simulink model "Quadcopter_v3_full"  (R2021a)
settings: Solver=ode4  StartTime=0.0  StopTime=87  FixedStep=0.001  RelTol=1e-6
values from neighbouring files (symbols this model uses):
  mean_wind = [2.72 , 1.75, -0.006]    [main_run.m]    (also in main_run_5_1.m; param_est.m = [2.72 , 1.75, .006])
  q = X(7:10)    [EKF_without_wind.m]
  r = linspace(floor(nr*0.01)/nr,1,nr)    [main_run.m]    (also in main_run_5_1.m)
  w1 = w(1)    [EKF_without_wind.m]
  x0 = [0,0,0,1,0,0,0,-P.mean_wind,0,0,0]    [main_run.m]    (also in main_run_5_1.m)
  xref = [1,1,-8,1,0,0,0,-P.mean_wind]    [main_run.m]    (also in main_run_5_1.m)
undefined symbols (not defined in the file or in its folder): HDBK, MIL, Moderate, P, u1, v1
libraries: simulink x1, aerolibwind2 x1
(part 1 of 5)
settings Model: PauseTimes=2  Creator=lab  LastModifiedBy=lab
settings DebuggingCC: ReadBeforeWriteMsg=EnableAllAsWarning  WriteAfterWriteMsg=EnableAllAsWarning  WriteAfterReadMsg=EnableAllAsWarning  SFMachineParentedDataDiag=warning
settings SFSimCC: SimTargetLang=C++

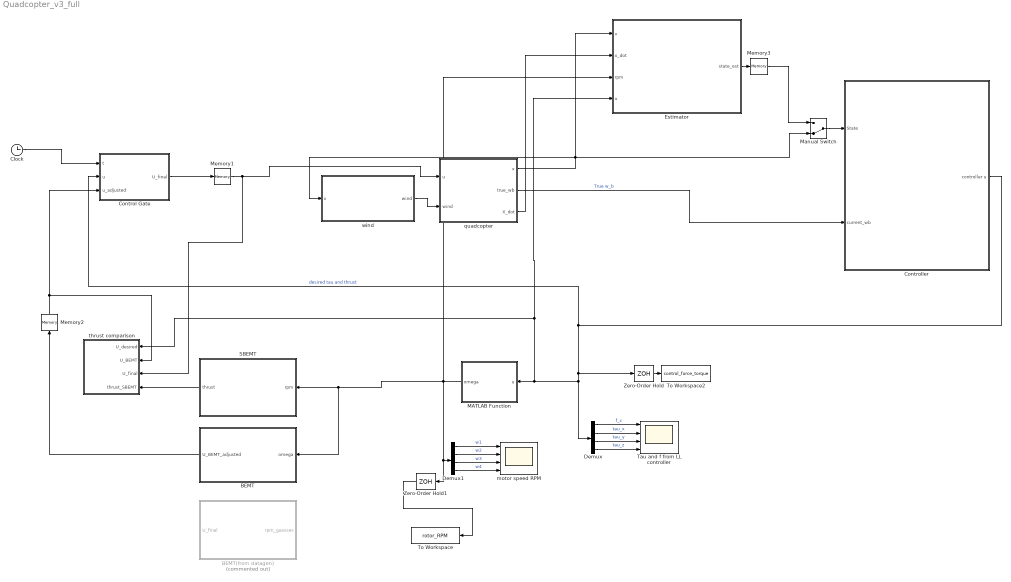
== system Quadcopter_v3_full ==
  BEMT : Subsystem
  BEMT(from datagen) : Subsystem  Commented=on
  Clock : Clock
  Control Gate : MATLAB Function  TreatAsAtomicUnit=on
  "Controller " : Subsystem
  Demux : Demux
  Demux1 : Demux
  Estimator : Subsystem
  MATLAB Function : MATLAB Function  TreatAsAtomicUnit=on
  Manual Switch : ManualSwitch  CurrentSetting=0
  Memory1 : Memory
  Memory2 : Memory
  Memory3 : Memory  InitialCondition=[0;0;0;1;0;0;0;0;0;0;0;0;0]
  SBEMT : Subsystem
  Tau and f from LL controller : Scope  NumInputPorts=4
  To Workspace : ToWorkspace  VariableName=rotor_RPM  SampleTime=-1
      settings: Save2DSignal=2-D array (concatenate along first dimension)
  To Workspace2 : ToWorkspace  VariableName=control_force_torque  SampleTime=-1
      settings: Save2DSignal=2-D array (concatenate along first dimension)
  Zero-Order Hold : ZeroOrderHold  SampleTime=0.01
  Zero-Order Hold1 : ZeroOrderHold  SampleTime=0.01
  motor speed RPM : Scope  NumInputPorts=4
  quadcopter : Subsystem
  thrust comparison : Subsystem
  wind : Subsystem
  wires:
  Zero-Order Hold/1 -> To Workspace2/1
  wind/1(wind) -> quadcopter/2(wind)
  Demux/1 -> Tau and f from LL controller/1  "f_c"
  Demux/2 -> Tau and f from LL controller/2  "tau_x"
  Demux/3 -> Tau and f from LL controller/3  "tau_y"
  Demux/4 -> Tau and f from LL controller/4  "tau_z"
  Demux1/2 -> motor speed RPM/2  "w2"
  Demux1/3 -> motor speed RPM/3  "w3"
  Demux1/4 -> motor speed RPM/4  "w4"
  Demux1/1 -> motor speed RPM/1  "w1"
  Zero-Order Hold1/1 -> To Workspace/1
  Control Gate/1(U_final) -> Memory1/1
  quadcopter/2(true_wb) -> "Controller "/2(current_wb)  "True w_b"
  quadcopter/3(X_dot) -> Estimator/2(x_dot)
  "Controller "/1(controller u) -> Demux/1, Estimator/4(u), thrust comparison/1(U_desired), MATLAB Function/1(u), Zero-Order Hold/1, Control Gate/2(u)  "desired tau and thrust"
  quadcopter/1(x) -> Estimator/1(x), Manual Switch/2, wind/1(x)
  MATLAB Function/1(omega) -> Estimator/3(rpm), BEMT/1(omega), SBEMT/1(rpm), Zero-Order Hold1/1, Demux1/1
  Memory1/1 -> thrust comparison/3(U_final), quadcopter/1(u)
  Clock/1 -> Control Gate/1(t)
  Memory2/1 -> thrust comparison/2(U_BEMT), Control Gate/3(u_adjusted)
  SBEMT/1(thrust) -> thrust comparison/4(thrust_SBEMT)
  BEMT/1(U_BEMT_adjusted) -> Memory2/1
  Estimator/1(state_est) -> Memory3/1
  Manual Switch/1 -> "Controller "/1(State)
  Memory3/1 -> Manual Switch/1

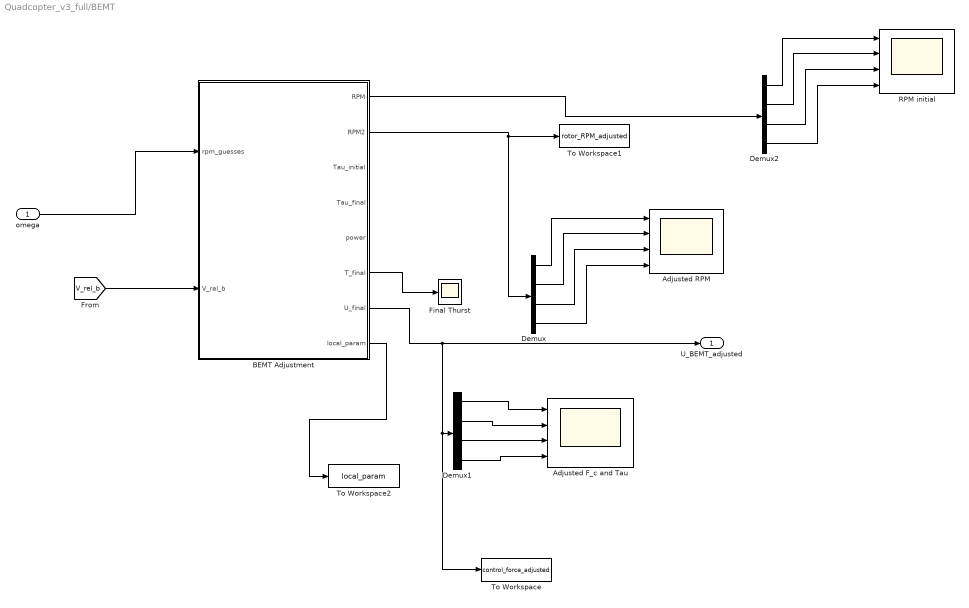
== system Quadcopter_v3_full/BEMT ==
  omega : Inport
  Adjusted F_c and Tau : Scope  NumInputPorts=4
  Adjusted RPM : Scope  NumInputPorts=4
  BEMT Adjustment : MATLAB Function  TreatAsAtomicUnit=on
  Demux : Demux
  Demux1 : Demux
  Demux2 : Demux
  Final Thurst : Scope
  RPM initial : Scope  NumInputPorts=4
  To Workspace : ToWorkspace  VariableName=control_force_adjusted  SampleTime=-1
      settings: Save2DSignal=2-D array (concatenate along first dimension)
  To Workspace1 : ToWorkspace  VariableName=rotor_RPM_adjusted  SampleTime=-1
      settings: Save2DSignal=2-D array (concatenate along first dimension)
  To Workspace2 : ToWorkspace  VariableName=local_param  SampleTime=-1
      settings: Save2DSignal=2-D array (concatenate along first dimension)
  U_BEMT_adjusted : Outport
  wires:
  omega/1 -> BEMT Adjustment/1(rpm_guesses)
  [V_rel_b] -> BEMT Adjustment/2(V_rel_b)
  BEMT Adjustment/2(RPM2) -> Demux/1, To Workspace1/1
  Demux/1 -> Adjusted RPM/1
  Demux/2 -> Adjusted RPM/2
  Demux/3 -> Adjusted RPM/3
  Demux/4 -> Adjusted RPM/4
  BEMT Adjustment/6(T_final) -> Final Thurst/1
  BEMT Adjustment/7(U_final) -> To Workspace/1, Demux1/1, U_BEMT_adjusted/1
  Demux1/1 -> Adjusted F_c and Tau/1
  Demux1/2 -> Adjusted F_c and Tau/2
  Demux1/3 -> Adjusted F_c and Tau/3
  Demux1/4 -> Adjusted F_c and Tau/4
  Demux2/1 -> RPM initial/1
  Demux2/4 -> RPM initial/4
  Demux2/3 -> RPM initial/3
  Demux2/2 -> RPM initial/2
  BEMT Adjustment/1(RPM) -> Demux2/1
  BEMT Adjustment/8(local_param) -> To Workspace2/1

== system Quadcopter_v3_full/BEMT(from datagen) ==
  rpm_guesses : Inport
  MATLAB Function1 : MATLAB Function  TreatAsAtomicUnit=on
  U_final : Outport
  wires:
  [V_rel_b] -> MATLAB Function1/2(V_rel_b)
  rpm_guesses/1 -> MATLAB Function1/1(rpm_guesses)
  MATLAB Function1/1(U_final) -> U_final/1

== system Quadcopter_v3_full/Controller  ==
  State : Inport
  current_wb : Inport  Port=2
  High Level Controller : Subsystem
  Low-Level Controller : Subsystem
      settings: PortSchema="{\"entries\":[{\"content\":{\"sides\":[{\"content\":{\"connectorIds\":[\"In1\"]},\"type\":\"ConnectorPlacement.EquallySpacedRectSide\",\"uuid\":\"a33d16ce-9843-4a8f-a539-e48e55dea327\"},{\"content\":{\"connectorIds\":[\"Out1\"],\"side\":\"RIGHT\"},\"type\":\"ConnectorPlacement.EquallySpacedRectSide\",\"uuid\":\"666ca801-6962-4f07-8037-ca18b43ecb76\"},{\"content\":{\"connectorIds\":[\"In2\"],\"side\":\"TOP\"},\"type\":\"ConnectorPlacement.EquallySpacedRectSide\",\"uuid\":\"a74aa88d-4aa1-42f8-8d8c-456156c6c0a0\"}]},\"type\":\"ConnectorPlacement.EquallySpacedConnector\",\"uuid\":\"b57d0f88-2cf0-4e3b-827d-8395103e5920\"}],\"packageUris\":[\"http://schema.mathworks.com/mf0/Connector/R2020b\"],\"version\":\"1.0\"}"
  To Workspace1 : ToWorkspace  VariableName=controller_omega  SampleTime=-1
      settings: Save2DSignal=2-D array (concatenate along first dimension)
  To Workspace5 : ToWorkspace  VariableName=states  SampleTime=-1
      settings: Save2DSignal=2-D array (concatenate along first dimension)
  Zero-Order Hold1 : ZeroOrderHold  SampleTime=0.01
  Zero-Order Hold2 : ZeroOrderHold  SampleTime=0.01
  controller u : Outport
  wires:
  State/1 -> High Level Controller/1(State), Zero-Order Hold2/1
  High Level Controller/1(" wx,wy,wz, f_c") -> Low-Level Controller/2(desired), Zero-Order Hold1/1  "desired w_b"
  current_wb/1 -> Low-Level Controller/1(prev_wb)
  Low-Level Controller/1(controller u) -> controller u/1  "desired tau and thrust"
  Zero-Order Hold2/1 -> To Workspace5/1
  Zero-Order Hold1/1 -> To Workspace1/1

== system Quadcopter_v3_full/Estimator ==
  x : Inport
  x_dot : Inport  Port=2
  rpm : Inport  Port=3
  u : Inport  Port=4
  Estimator : Subsystem
  To Workspace : ToWorkspace  VariableName=state_estimate  SampleTime=-1
      settings: Save2DSignal=2-D array (concatenate along first dimension)
  sensors : Subsystem
  state_est_aug : MATLAB Function  TreatAsAtomicUnit=on
  state_est : Outport
  wires:
  x/1 -> Estimator/5(X), sensors/1(x)
  sensors/1(GPS) -> Estimator/1(GPS)
  sensors/3(B_b) -> Estimator/3(B_b)
  rpm/1 -> Estimator/4(rpm)
  x_dot/1 -> sensors/2(x_dot)
  sensors/2(Accel_Gyro) -> state_est_aug/2(accel_gyro), Estimator/2(Accel_Gyro)
  u/1 -> Estimator/6(f_c)
  Estimator/1(state_est) -> state_est_aug/1(states_est), To Workspace/1
  state_est_aug/1(y) -> state_est/1

== system Quadcopter_v3_full/SBEMT ==
  rpm : Inport
  Simplified BEMT : MATLAB Function  TreatAsAtomicUnit=on
  thrust : Outport
  wires:
  rpm/1 -> Simplified BEMT/2(rpm)
  Simplified BEMT/1(Y) -> thrust/1  "SBEM f_c"
  [V_rel_b] -> Simplified BEMT/1(V_rb)

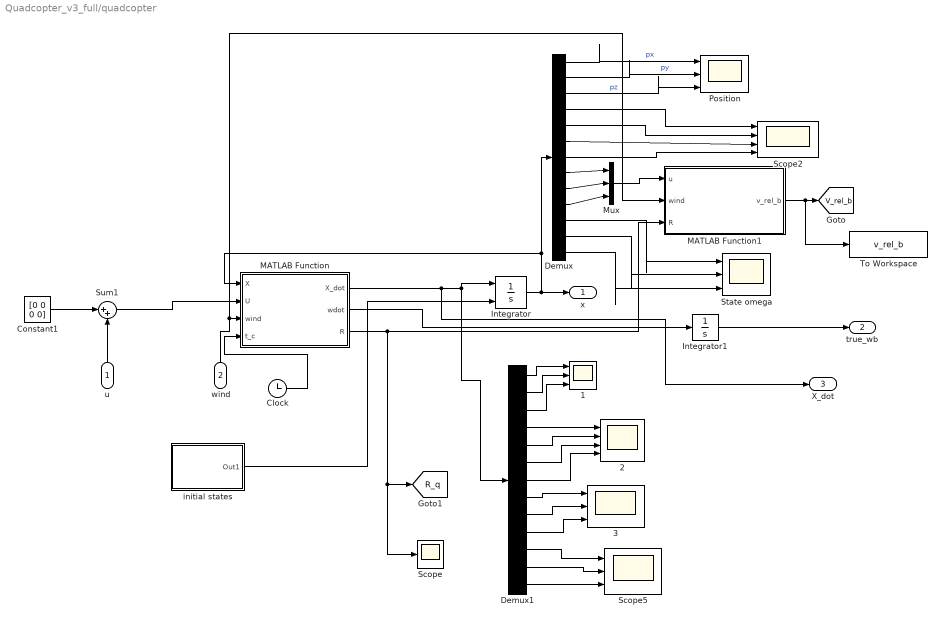
== system Quadcopter_v3_full/quadcopter ==
  u : Inport
  wind : Inport  Port=2
  1 : Scope  NumInputPorts=3
  2 : Scope  NumInputPorts=4
  3 : Scope  NumInputPorts=3
  Clock : Clock
  Constant1 : Constant  Value=[0 0 0 0]
  Demux : Demux  Outputs=13
  Demux1 : Demux  Outputs=13
  Integrator : Integrator  InitialConditionSource=external
  Integrator1 : Integrator  InitialCondition=[0,0,0]
  MATLAB Function : MATLAB Function  TreatAsAtomicUnit=on
  MATLAB Function1 : MATLAB Function  TreatAsAtomicUnit=on
  Mux : Mux  Inputs=3
  Position : Scope  NumInputPorts=3
  Scope : Scope
  Scope2 : Scope  NumInputPorts=4
  Scope5 : Scope  NumInputPorts=3
  State omega : Scope  NumInputPorts=3
  Sum1 : Sum  Inputs=|++
  To Workspace : ToWorkspace  VariableName=v_rel_b  SampleTime=-1
      settings: Save2DSignal=2-D array (concatenate along first dimension)
  initial states : Subsystem
  x : Outport
  true_wb : Outport  Port=2  OutDataTypeStr=double
  X_dot : Outport  Port=3
  tag scope: R_q=global, V_rel_b=global
  wires:
  Integrator/1 -> x/1, Demux/1, MATLAB Function/1(X)
  u/1 -> Sum1/2
  Sum1/1 -> MATLAB Function/2(U)
  Constant1/1 -> Sum1/1
  Demux1/6 -> 2/3
  Demux1/2 -> 1/2
  Demux1/5 -> 2/2
  Demux1/4 -> 2/1
  Demux1/3 -> 1/3
  Demux1/1 -> 1/1
  MATLAB Function/1(X_dot) -> X_dot/1, Integrator/1, Demux1/1
  wind/1 -> MATLAB Function1/2(wind), MATLAB Function/3(wind)
  initial states/1(Out1) -> Integrator/2
  Demux1/7 -> 2/4
  Demux1/8 -> 3/1
  Demux1/9 -> 3/2
  Demux1/10 -> 3/3
  Demux/1 -> Position/1  "px"
  Demux/2 -> Position/2  "py"
  Demux/3 -> Position/3  "pz"
  Demux/4 -> Scope2/1
  Demux/5 -> Scope2/2
  Demux/6 -> Scope2/3
  Demux/7 -> Scope2/4
  Demux1/11 -> Scope5/1
  Demux1/12 -> Scope5/2
  Demux1/13 -> Scope5/3
  MATLAB Function/2(wdot) -> Integrator1/1
  Demux/11 -> State omega/1
  Demux/12 -> State omega/2
  Demux/13 -> State omega/3
  Integrator1/1 -> true_wb/1
  Demux/8 -> Mux/1
  Demux/9 -> Mux/2
  Demux/10 -> Mux/3
  Mux/1 -> MATLAB Function1/1(u)
  MATLAB Function1/1(v_rel_b) -> To Workspace/1, [V_rel_b]
  MATLAB Function/3(R) -> Scope/1, [R_q], MATLAB Function1/3(R)
  Clock/1 -> MATLAB Function/4(t_c)

== system Quadcopter_v3_full/thrust comparison ==
  U_desired : Inport
  U_BEMT : Inport  Port=2
  U_final : Inport  Port=3
  thrust_SBEMT : Inport  Port=4
  Add : Sum  Inputs=+-
  Demux : Demux
  Demux1 : Demux
  Demux2 : Demux
  Scope : Scope  NumInputPorts=4
  Scope1 : Scope
  To Workspace : ToWorkspace  VariableName=thrust_desired  SampleTime=-1
      settings: Save2DSignal=2-D array (concatenate along first dimension)
  To Workspace1 : ToWorkspace  VariableName=thrust_BEMT  SampleTime=-1
      settings: Save2DSignal=2-D array (concatenate along first dimension)
  To Workspace2 : ToWorkspace  VariableName=thrust_final  SampleTime=-1
      settings: Save2DSignal=2-D array (concatenate along first dimension)
  To Workspace3 : ToWorkspace  VariableName=thrust_SBEMT  SampleTime=-1
      settings: Save2DSignal=2-D array (concatenate along first dimension)
  wires:
  U_desired/1 -> Demux/1
  U_BEMT/1 -> Demux1/1
  U_final/1 -> Demux2/1
  Demux/1 -> To Workspace/1, Scope/1  "thrust_desired"
  Demux1/1 -> To Workspace1/1, Scope/2  "thrust_BEMT"
  Demux2/1 -> Add/2, To Workspace2/1, Scope/3  "thrust_final"
  thrust_SBEMT/1 -> Add/1, To Workspace3/1, Scope/4  "thrust_SBEMT"
  Add/1 -> Scope1/1

== system Quadcopter_v3_full/wind ==
  x : Inport
  Constant_Wind : Subsystem
  Demux : Demux  Outputs=3
  Dryden Wind : Subsystem  Commented=on
  LES_wind : Subsystem  Commented=on
  Manual Switch : ManualSwitch
  To Workspace4 : ToWorkspace  VariableName=Wind  SampleTime=-1
      settings: Save2DSignal=2-D array (concatenate along first dimension)
  Zero-Order Hold1 : ZeroOrderHold  SampleTime=0.01
  sinusoidal_wind : Subsystem  Commented=on
  wind_vel : Scope  NumInputPorts=3
  wind : Outport
  wires:
  Manual Switch/1 -> Zero-Order Hold1/1, Demux/1, wind/1
  Constant_Wind/1(y) -> Manual Switch/1
  Zero-Order Hold1/1 -> To Workspace4/1
  LES_wind/1(Out1) -> Manual Switch/2
  x/1 -> LES_wind/1(x)
  Demux/1 -> wind_vel/1
  Demux/2 -> wind_vel/2
  Demux/3 -> wind_vel/3

== system Quadcopter_v3_full/Controller /High Level Controller ==
  State : Inport
  Clock : Clock
  Demux : Demux
  RS Controller : MATLAB Function  InitFcn="run(\"get_finitegain.m\")"  TreatAsAtomicUnit=on  SystemSampleTime=.05
  omega and fc from HL controller : Scope  NumInputPorts=4
  trajectory : Subsystem
  " wx,wy,wz, f_c" : Outport
  wires:
  RS Controller/1(y) -> " wx,wy,wz, f_c"/1, Demux/1
  trajectory/1(Out1) -> RS Controller/2(r)
  Demux/4 -> omega and fc from HL controller/4  "f_c"
  Demux/2 -> omega and fc from HL controller/2  "wy"
  Demux/1 -> omega and fc from HL controller/1  "wx"
  Demux/3 -> omega and fc from HL controller/3  "wz"
  State/1 -> RS Controller/1(x), trajectory/1(X)
  Clock/1 -> RS Controller/3(t)

== system Quadcopter_v3_full/Controller /Low-Level Controller ==
  prev_wb : Inport
  desired : Inport  Port=2
  Low level controller : MATLAB Function  TreatAsAtomicUnit=on  SystemSampleTime=.005
  controller u : Outport
  wires:
  Low level controller/1(u) -> controller u/1
  desired/1 -> Low level controller/2(desired)
  prev_wb/1 -> Low level controller/1(true_u)

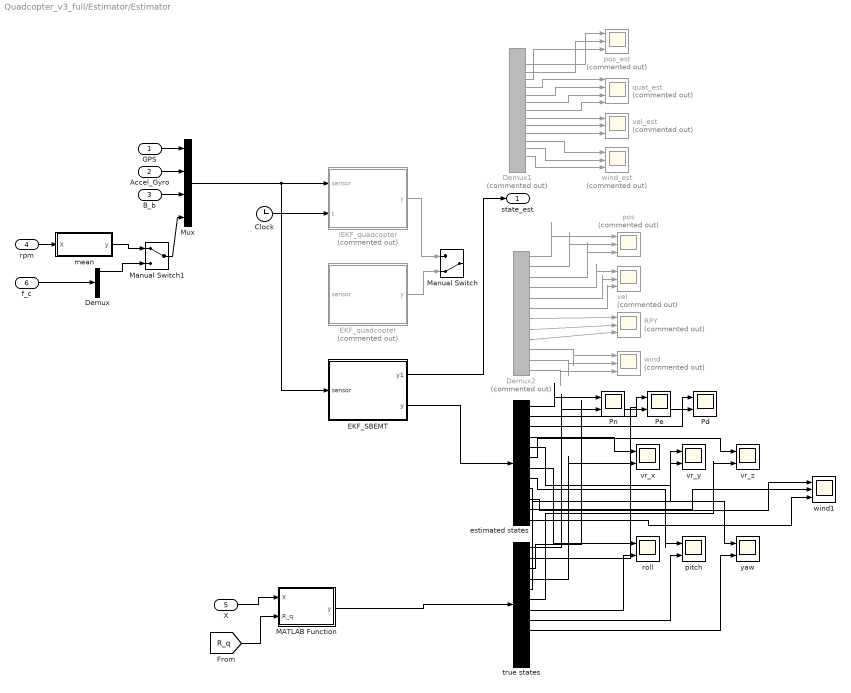
== system Quadcopter_v3_full/Estimator/Estimator ==
  GPS : Inport
  Accel_Gyro : Inport  Port=2
  B_b : Inport  Port=3
  rpm : Inport  Port=4
  X : Inport  Port=5
  f_c : Inport  Port=6
  Clock : Clock
  Demux : Demux
  Demux1 : Demux  Commented=on  Outputs=13
  Demux2 : Demux  Commented=on  Outputs=12
  EKF_SBEMT : MATLAB Function  InitFcn=addpath('quaternion_library');  TreatAsAtomicUnit=on  SystemSampleTime=0.01
  EKF_quadcopter : MATLAB Function  Commented=on  InitFcn=addpath('quaternion_library');  TreatAsAtomicUnit=on  SystemSampleTime=0.01
  IEKF_quadcopter : MATLAB Function  Commented=on  InitFcn=addpath('quaternion_library');  TreatAsAtomicUnit=on  SystemSampleTime=0.01
  MATLAB Function : MATLAB Function  TreatAsAtomicUnit=on
  Manual Switch : ManualSwitch  CurrentSetting=0
  Manual Switch1 : ManualSwitch
  Mux : Mux
  Pd : Scope  NumInputPorts=2
  Pe : Scope  NumInputPorts=2
  Pn : Scope  NumInputPorts=2
  RPY : Scope  Commented=on  NumInputPorts=3
  estimated states : Demux  Outputs=12
  mean : MATLAB Function  TreatAsAtomicUnit=on
  pitch : Scope  NumInputPorts=2
  pos : Scope  Commented=on  NumInputPorts=3
  pos_est : Scope  Commented=on  NumInputPorts=3
  quat_est : Scope  Commented=on  NumInputPorts=4
  roll : Scope  NumInputPorts=2
  true states : Demux  Outputs=12
  vel : Scope  Commented=on  NumInputPorts=3
  vel_est : Scope  Commented=on  NumInputPorts=3
  vr_x : Scope  NumInputPorts=2
  vr_y : Scope  NumInputPorts=2
  vr_z : Scope  NumInputPorts=2
  wind : Scope  Commented=on  NumInputPorts=3
  wind1 : Scope  NumInputPorts=3
  wind_est : Scope  Commented=on  NumInputPorts=3
  yaw : Scope  NumInputPorts=2
  state_est : Outport
  wires:
  GPS/1 -> Mux/1
  Accel_Gyro/1 -> Mux/2
  B_b/1 -> Mux/3
  rpm/1 -> mean/1(X)
  Demux1/1 -> pos_est/1
  Demux1/2 -> pos_est/2
  Demux1/3 -> pos_est/3
  Demux1/4 -> quat_est/1
  Demux1/5 -> quat_est/2
  Demux1/6 -> quat_est/3
  Demux1/7 -> quat_est/4
  Demux1/8 -> vel_est/1
  Demux1/9 -> vel_est/2
  Demux1/10 -> vel_est/3
  Demux1/11 -> wind_est/1
  Demux1/12 -> wind_est/2
  Demux1/13 -> wind_est/3
  Demux2/6 -> vel/3
  Demux2/5 -> vel/2
  Demux2/1 -> pos/1
  Demux2/2 -> pos/2
  Demux2/4 -> vel/1
  Demux2/3 -> pos/3
  Demux2/7 -> RPY/1
  Demux2/8 -> RPY/2
  Demux2/9 -> RPY/3
  Demux2/10 -> wind/1
  Demux2/11 -> wind/2
  Demux2/12 -> wind/3
  IEKF_quadcopter/1(y) -> Manual Switch/1
  X/1 -> MATLAB Function/1(X)
  estimated states/1 -> Pn/1
  true states/1 -> Pn/2
  estimated states/2 -> Pe/1
  true states/2 -> Pe/2
  estimated states/3 -> Pd/1
  true states/3 -> Pd/2
  estimated states/4 -> vr_x/1
  true states/4 -> vr_x/2
  estimated states/5 -> vr_y/1
  true states/5 -> vr_y/2
  estimated states/6 -> vr_z/1
  true states/6 -> vr_z/2
  estimated states/7 -> roll/1
  true states/7 -> roll/2
  estimated states/8 -> pitch/1
  true states/8 -> pitch/2
  estimated states/9 -> yaw/1
  true states/9 -> yaw/2
  MATLAB Function/1(y) -> true states/1
  estimated states/10 -> wind1/1
  estimated states/11 -> wind1/2
  estimated states/12 -> wind1/3
  Clock/1 -> IEKF_quadcopter/2(t)
  Mux/1 -> EKF_SBEMT/1(sensor), IEKF_quadcopter/1(sensor)
  Manual Switch1/1 -> Mux/4
  mean/1(y) -> Manual Switch1/1
  f_c/1 -> Demux/1
  Demux/1 -> Manual Switch1/2
  EKF_quadcopter/1(y) -> Manual Switch/2
  [R_q] -> MATLAB Function/2(R_q)
  EKF_SBEMT/2(y) -> estimated states/1
  EKF_SBEMT/1(y1) -> state_est/1

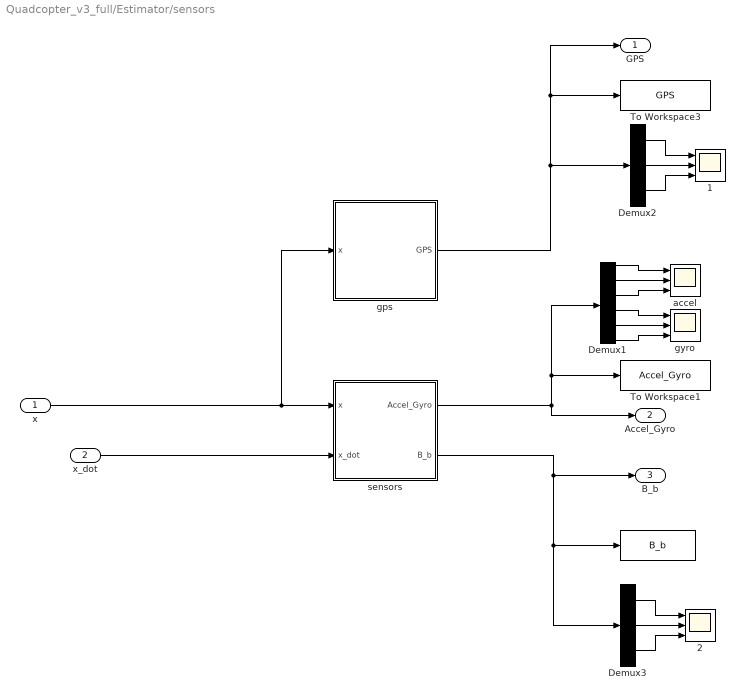
== system Quadcopter_v3_full/Estimator/sensors ==
  x : Inport
  x_dot : Inport  Port=2
  " " : ToWorkspace  VariableName=B_b  SampleTime=-1
      settings: Save2DSignal=2-D array (concatenate along first dimension)
  1 : Scope  NumInputPorts=3
  2 : Scope  NumInputPorts=3
  Demux1 : Demux  Outputs=6
  Demux2 : Demux  Outputs=3
  Demux3 : Demux  Outputs=3
  To Workspace1 : ToWorkspace  VariableName=Accel_Gyro  SampleTime=-1
      settings: Save2DSignal=2-D array (concatenate along first dimension)
  To Workspace3 : ToWorkspace  VariableName=GPS  SampleTime=-1
      settings: Save2DSignal=2-D array (concatenate along first dimension)
  accel : Scope  NumInputPorts=3
  gps : MATLAB Function  TreatAsAtomicUnit=on  SystemSampleTime=P.Ts_gps
  gyro : Scope  NumInputPorts=3
  sensors : MATLAB Function  TreatAsAtomicUnit=on  SystemSampleTime=P.Ts_gy_ac
  GPS : Outport
  Accel_Gyro : Outport  Port=2
  B_b : Outport  Port=3
  wires:
  Demux2/2 -> 1/2
  sensors/2(B_b) -> Demux3/1, " "/1, B_b/1
  Demux1/2 -> accel/2
  Demux3/2 -> 2/2
  Demux3/3 -> 2/3
  Demux2/3 -> 1/3
  x/1 -> sensors/1(x), gps/1(x)
  sensors/1(Accel_Gyro) -> Accel_Gyro/1, Demux1/1, To Workspace1/1
  gps/1(GPS) -> GPS/1, To Workspace3/1, Demux2/1
  Demux3/1 -> 2/1
  Demux1/3 -> accel/3
  Demux1/5 -> gyro/2
  Demux1/1 -> accel/1
  Demux1/4 -> gyro/1
  Demux1/6 -> gyro/3
  Demux2/1 -> 1/1
  x_dot/1 -> sensors/2(x_dot)

== system Quadcopter_v3_full/quadcopter/initial states ==
  Constant : Constant  Value=x0
  MATLAB Function1 : MATLAB Function  Commented=on  TreatAsAtomicUnit=on
  To Workspace4 : ToWorkspace  VariableName=X0  SampleTime=-1
  Out1 : Outport
  wires:
  Constant/1 -> To Workspace4/1, Out1/1

== system Quadcopter_v3_full/wind/Constant_Wind ==
  wind1 : Constant  Value=mean_wind
  y : Outport
  wires:
  wind1/1 -> y/1

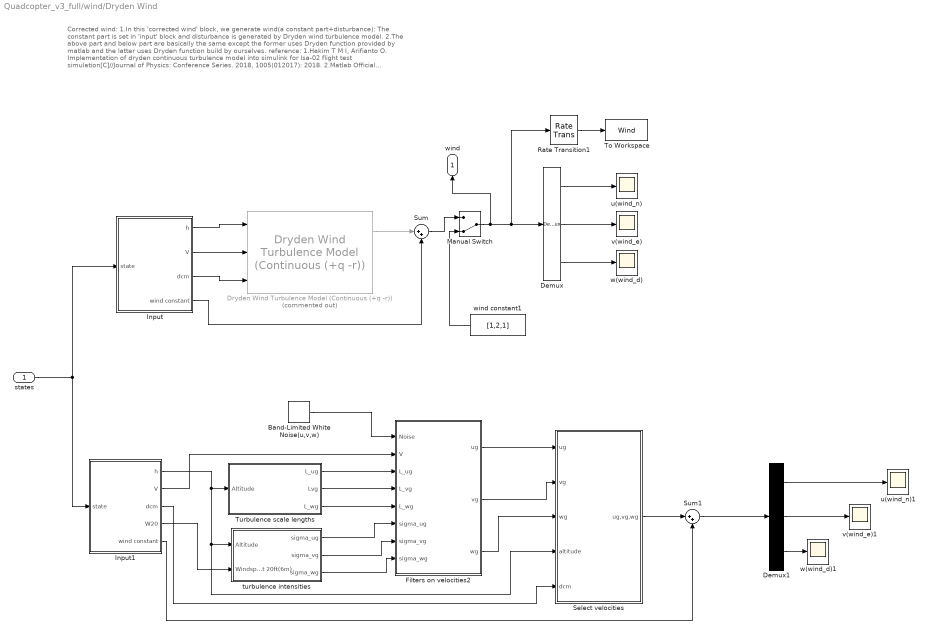
== system Quadcopter_v3_full/wind/Dryden Wind ==
  note: Corrected wind:
      | 1.In this 'corrected wind' block, we generate wind(a constant part+disturbance): The constant part is set in 'input' block and disturbance is generated by Dryden wind turbulence model.
      |
      | 2.The above part and below part are basically the same except the former uses Dryden function provided by matlab and the latter uses Dryden function build by ourselves.
      |
      | reference:
      | 1.Hakim T M I, Arifianto O. Implementation of dryden continuous turbulence model into simulink for lsa-02 flight test simulation[C]//Journal of Physics: Conference Series. 2018, 1005(012017): 2018.
      | 2.Matlab Official documents about Dryden Wind Turbulence Model
  states : Inport
  Band-Limited White Noise(u,v,w) : simulink/Sources/Band-Limited White Noise  Cov=[1 1 1]*pi  Ts=0.1  seed=[23341 23342 23343]
  Demux : Demux  Outputs=3
  Demux1 : Demux  Outputs=3
  Dryden Wind Turbulence Model (Continuous (+q -r)) : aerolibwind2/Dryden Wind Turbulence Model  (Continuous (+q -r))  Commented=on  units=Metric (MKS)  spec=MIL-HDBK-1797  model=Continuous Dryden (-q +r)  W20=15  Wdeg=45  TurbProb=10^-3 - Moderate  L_high=533.4  Wingspan=0.4  ts=0.1  Seed=[23341 23342 23343 23344]  T_on=on
  Filters on velocities2 : Subsystem
  Input : Subsystem
  Input1 : Subsystem
  Manual Switch : ManualSwitch  CurrentSetting=0
  Rate Transition1 : RateTransition  OutPortSampleTime=0.01
  Select velocities : Subsystem
  Sum : Sum  Inputs=|++
  Sum1 : Sum  Inputs=|++
  To Workspace : ToWorkspace  VariableName=Wind  SaveFormat=Timeseries  SampleTime=-1
  Turbulence scale lengths : Subsystem
  turbulence intensities : Subsystem
  u(wind_n) : Scope
  u(wind_n)1 : Scope
  v(wind_e) : Scope
  v(wind_e)1 : Scope
  w(wind_d) : Scope
  w(wind_d)1 : Scope
  wind constant1 : Constant  Value=[1,2,1]
  wind : Outport
  wires:
  Input/1(h) -> Dryden Wind Turbulence Model (Continuous (+q -r))/1
  Input/2(V) -> Dryden Wind Turbulence Model (Continuous (+q -r))/2
  Input/3(dcm) -> Dryden Wind Turbulence Model (Continuous (+q -r))/3
  states/1 -> Input/1(state), Input1/1(state)
  Dryden Wind Turbulence Model (Continuous (+q -r))/1 -> Sum/1
  Input1/1(h) -> Turbulence scale lengths/1(Altitude), turbulence intensities/1(Altitude), Select velocities/4(altitude)
  Input1/4(W20) -> turbulence intensities/2(Windspeed at 20ft(6m))
  turbulence intensities/2(sigma_vg) -> Filters on velocities2/7(sigma_vg)
  turbulence intensities/3(sigma_wg) -> Filters on velocities2/8(sigma_wg)
  Turbulence scale lengths/1(L_ug) -> Filters on velocities2/3(L_ug)
  Turbulence scale lengths/2(Lvg) -> Filters on velocities2/4(L_vg)
  Turbulence scale lengths/3(L_wg) -> Filters on velocities2/5(L_wg)
  Band-Limited White Noise(u,v,w)/1 -> Filters on velocities2/1(Noise)
  Input1/2(V) -> Filters on velocities2/2(V)
  turbulence intensities/1(sigma_ug) -> Filters on velocities2/6(sigma_ug)
  Filters on velocities2/1(ug) -> Select velocities/1(ug)
  Filters on velocities2/2(vg) -> Select velocities/2(vg)
  Filters on velocities2/3(wg) -> Select velocities/3(wg)
  Input1/3(dcm) -> Select velocities/5(dcm)
  Demux/1 -> u(wind_n)/1
  Demux/2 -> v(wind_e)/1
  Demux/3 -> w(wind_d)/1
  Input/4(wind constant) -> Sum/2
  Demux1/1 -> u(wind_n)1/1
  Demux1/2 -> v(wind_e)1/1
  Demux1/3 -> w(wind_d)1/1
  Input1/5(wind constant) -> Sum1/2
  Select velocities/1(ug,vg,wg) -> Sum1/1
  Sum1/1 -> Demux1/1
  Manual Switch/1 -> Rate Transition1/1, Demux/1, wind/1
  Sum/1 -> Manual Switch/1
  wind constant1/1 -> Manual Switch/2
  Rate Transition1/1 -> To Workspace/1

== system Quadcopter_v3_full/wind/LES_wind ==
  x : Inport
  Clock : Clock
  Constant : Constant  Value=u1
  Constant1 : Constant  Value=v1
  Constant2 : Constant  Value=w1
  From Workspace : FromWorkspace  Commented=on  VariableName=LES_wind_8m  SampleTime=-1
  From Workspace1 : FromWorkspace  VariableName=LES_wind  SampleTime=1
  MATLAB Function : MATLAB Function  TreatAsAtomicUnit=on
  Manual Switch1 : ManualSwitch
  Out1 : Outport
  wires:
  Manual Switch1/1 -> Out1/1
  x/1 -> MATLAB Function/1(x)
  Clock/1 -> MATLAB Function/2(t)
  Constant/1 -> MATLAB Function/3(u_wind)
  Constant1/1 -> MATLAB Function/4(v_wind)
  Constant2/1 -> MATLAB Function/5(w_wind)
  From Workspace1/1 -> Manual Switch1/1
  MATLAB Function/1(wind_vel) -> Manual Switch1/2

== system Quadcopter_v3_full/wind/sinusoidal_wind ==
  Clock : Clock
  From Workspace : FromWorkspace  VariableName=LES_wind_8m  SampleTime=-1
  Scope : Scope
  To Workspace4 : ToWorkspace  VariableName=Wind  SaveFormat=Timeseries  SampleTime=-1
  Zero-Order Hold1 : ZeroOrderHold  SampleTime=0.01
  sinusoidal part : MATLAB Function  TreatAsAtomicUnit=on
  y : Outport
  wires:
  From Workspace/1 -> sinusoidal part/1(LES)
  Clock/1 -> sinusoidal part/2(t)
  Zero-Order Hold1/1 -> To Workspace4/1
  sinusoidal part/1(y) -> Zero-Order Hold1/1, Scope/1, y/1

== system Quadcopter_v3_full/Controller /High Level Controller/trajectory ==
  X : Inport
  Clock : Clock
  "Desired Position, quat and velocity " : Constant  Value=xref
  MATLAB Function : MATLAB Function  TreatAsAtomicUnit=on
  Manual Switch : ManualSwitch  CurrentSetting=0
  circle_traj : MATLAB Function  Commented=on  TreatAsAtomicUnit=on
  squre_traj : MATLAB Function  Commented=on  TreatAsAtomicUnit=on
  Out1 : Outport
  wires:
  Manual Switch/1 -> Out1/1
  "Desired Position, quat and velocity "/1 -> Manual Switch/1
  X/1 -> squre_traj/1(X)
  Clock/1 -> MATLAB Function/1(t)
  MATLAB Function/1(xdes) -> Manual Switch/2

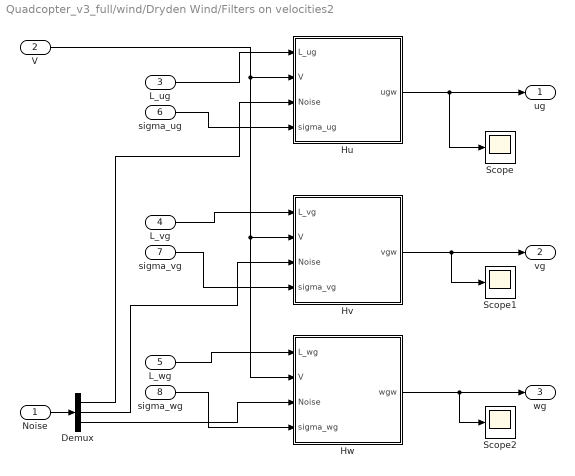
== system Quadcopter_v3_full/wind/Dryden Wind/Filters on velocities2 ==
  Noise : Inport
  V : Inport  Port=2
  L_ug : Inport  Port=3
  L_vg : Inport  Port=4
  L_wg : Inport  Port=5
  sigma_ug : Inport  Port=6
  sigma_vg : Inport  Port=7
  sigma_wg : Inport  Port=8
  Demux : Demux  Outputs=3
  Hu : Subsystem
  Hv : Subsystem
  Hw : Subsystem
  Scope : Scope
  Scope1 : Scope
  Scope2 : Scope
  ug : Outport
  vg : Outport  Port=2
  wg : Outport  Port=3
  wires:
  Noise/1 -> Demux/1
  V/1 -> Hw/2(V), Hv/2(V), Hu/2(V)
  L_ug/1 -> Hu/1(L_ug)
  sigma_ug/1 -> Hu/4(sigma_ug)
  Hu/1(ugw) -> Scope/1, ug/1
  L_vg/1 -> Hv/1(L_vg)
  sigma_vg/1 -> Hv/4(sigma_vg)
  Hv/1(vgw) -> Scope1/1, vg/1
  L_wg/1 -> Hw/1(L_wg)
  Demux/1 -> Hu/3(Noise)
  Demux/2 -> Hv/3(Noise)
  Demux/3 -> Hw/3(Noise)
  sigma_wg/1 -> Hw/4(sigma_wg)
  Hw/1(wgw) -> Scope2/1, wg/1

== system Quadcopter_v3_full/wind/Dryden Wind/Input ==
  state : Inport
  Abs : Abs
  DCM/rotation matrix : MATLAB Function  TreatAsAtomicUnit=on
  Demux : Demux  Outputs=12
  MATLAB Function : MATLAB Function  TreatAsAtomicUnit=on
  Mux : Mux  Inputs=9
  Mux1 : Mux  Inputs=3
  Scope : Scope
  Terminator : Terminator
  wind : Constant  Value=[0.1,0.1,0]
  h : Outport
  V : Outport  Port=2
  dcm : Outport  Port=3
  wind constant : Outport  Port=4
  wires:
  state/1 -> DCM/rotation matrix/1(x), Demux/1
  DCM/rotation matrix/1(R) -> dcm/1
  Mux/1 -> Terminator/1
  Demux/1 -> Mux/1
  MATLAB Function/1(V) -> Scope/1, V/1
  Demux/4 -> Mux1/1
  Demux/5 -> Mux1/2
  Demux/6 -> Mux1/3
  Demux/2 -> Mux/2
  Demux/3 -> Abs/1, Mux/3
  Demux/7 -> Mux/4
  Demux/8 -> Mux/5
  Demux/9 -> Mux/6
  Demux/10 -> Mux/7
  Demux/11 -> Mux/8
  Demux/12 -> Mux/9
  wind/1 -> wind constant/1, MATLAB Function/1(wind)
  Mux1/1 -> MATLAB Function/2(vel)
  Abs/1 -> h/1

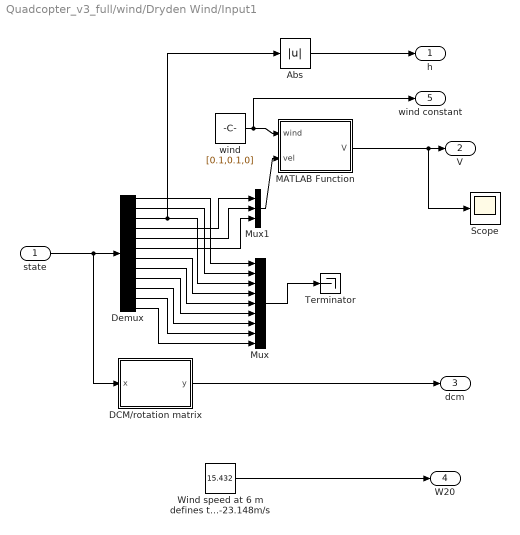
== system Quadcopter_v3_full/wind/Dryden Wind/Input1 ==
  state : Inport
  Abs : Abs
  DCM/rotation matrix : MATLAB Function  TreatAsAtomicUnit=on
  Demux : Demux  Outputs=12
  MATLAB Function : MATLAB Function  TreatAsAtomicUnit=on
  Mux : Mux  Inputs=9
  Mux1 : Mux  Inputs=3
  Scope : Scope
  Terminator : Terminator
  Wind speed at 6 m defines the low-altitude intensity (m/s) Light-7.716m/s Moderate-15.432m/s Severe-23.148m/s : Constant  Value=15.432
  wind : Constant  Value=[0.1,0.1,0]
  h : Outport
  V : Outport  Port=2
  dcm : Outport  Port=3
  W20 : Outport  Port=4
  wind constant : Outport  Port=5
  wires:
  state/1 -> DCM/rotation matrix/1(x), Demux/1
  DCM/rotation matrix/1(y) -> dcm/1
  Mux/1 -> Terminator/1
  Demux/1 -> Mux/1
  MATLAB Function/1(V) -> Scope/1, V/1
  Demux/4 -> Mux1/1
  Demux/5 -> Mux1/2
  Demux/6 -> Mux1/3
  Demux/2 -> Mux/2
  Demux/3 -> Abs/1, Mux/3
  Demux/7 -> Mux/4
  Demux/8 -> Mux/5
  Demux/9 -> Mux/6
  Demux/10 -> Mux/7
  Demux/11 -> Mux/8
  Demux/12 -> Mux/9
  wind/1 -> wind constant/1, MATLAB Function/1(wind)
  Mux1/1 -> MATLAB Function/2(vel)
  Wind speed at 6 m defines the low-altitude intensity (m/s) Light-7.716m/s Moderate-15.432m/s Severe-23.148m/s/1 -> W20/1
  Abs/1 -> h/1

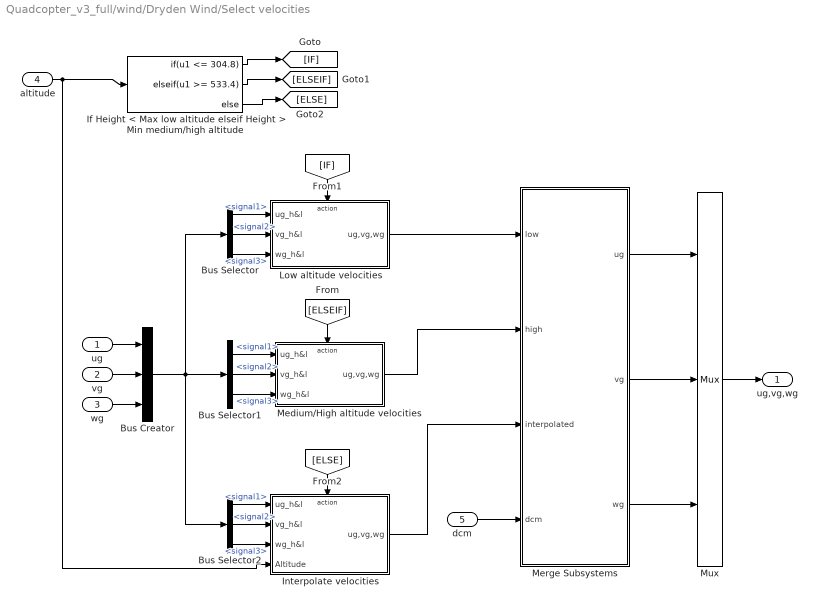
== system Quadcopter_v3_full/wind/Dryden Wind/Select velocities ==
  ug : Inport
  vg : Inport  Port=2
  wg : Inport  Port=3
  altitude : Inport  Port=4
  dcm : Inport  Port=5
  Bus Creator : BusCreator  Inputs=3
  Bus Selector : BusSelector  OutputSignals=signal1,signal2,signal3
  Bus Selector1 : BusSelector  OutputSignals=signal1,signal2,signal3
  Bus Selector2 : BusSelector  OutputSignals=signal1,signal2,signal3
  If Height < Max low altitude elseif Height > Min medium/high altitude : If  IfExpression=u1 <= 304.8  ElseIfExpressions=u1 >= 533.4
  Interpolate velocities : Subsystem  TreatAsAtomicUnit=on
  "Low altitude velocities " : Subsystem  TreatAsAtomicUnit=on
  Medium/High altitude velocities : Subsystem  TreatAsAtomicUnit=on
  Merge Subsystems : Subsystem
  Mux : Mux  Inputs=3
  ug,vg,wg : Outport
  wires:
  altitude/1 -> Interpolate velocities/4(Altitude), If Height < Max low altitude elseif Height > Min medium/high altitude/1
  If Height < Max low altitude elseif Height > Min medium/high altitude/1 -> [IF]
  If Height < Max low altitude elseif Height > Min medium/high altitude/2 -> [ELSEIF]
  [ELSEIF] -> Medium/High altitude velocities/Action
  "Low altitude velocities "/1(ug,vg,wg) -> Merge Subsystems/1(low)
  [IF] -> "Low altitude velocities "/Action
  Interpolate velocities/1(ug,vg,wg) -> Merge Subsystems/3(interpolated)
  [ELSE] -> Interpolate velocities/Action
  dcm/1 -> Merge Subsystems/4(dcm)
  vg/1 -> Bus Creator/2
  wg/1 -> Bus Creator/3
  ug/1 -> Bus Creator/1
  Bus Creator/1 -> Bus Selector2/1, Bus Selector1/1, Bus Selector/1
  Bus Selector2/1 -> Interpolate velocities/1(ug_h&l)  "<signal1>"
  Bus Selector2/2 -> Interpolate velocities/2(vg_h&l)  "<signal2>"
  Bus Selector2/3 -> Interpolate velocities/3(wg_h&l)  "<signal3>"
  Bus Selector/1 -> "Low altitude velocities "/1(ug_h&l)  "<signal1>"
  Bus Selector/2 -> "Low altitude velocities "/2(vg_h&l)  "<signal2>"
  Bus Selector/3 -> "Low altitude velocities "/3(wg_h&l)  "<signal3>"
  Bus Selector1/1 -> Medium/High altitude velocities/1(ug_h&l)  "<signal1>"
  Bus Selector1/2 -> Medium/High altitude velocities/2(vg_h&l)  "<signal2>"
  Bus Selector1/3 -> Medium/High altitude velocities/3(wg_h&l)  "<signal3>"
  If Height < Max low altitude elseif Height > Min medium/high altitude/3 -> [ELSE]
  Medium/High altitude velocities/1(ug,vg,wg) -> Merge Subsystems/2(high)
  Merge Subsystems/2(vg) -> Mux/2
  Merge Subsystems/1(ug) -> Mux/1
  Merge Subsystems/3(wg) -> Mux/3
  Mux/1 -> ug,vg,wg/1

== system Quadcopter_v3_full/wind/Dryden Wind/Turbulence scale lengths ==
  Altitude : Inport
  Low altitude scale length : Subsystem
  Medium/High altitude scale length : Subsystem
  Mux : Mux  Inputs=2
  Mux1 : Mux  Inputs=2
  Mux2 : Mux  Inputs=2
  L_ug : Outport
  Lvg : Outport  Port=2
  L_wg : Outport  Port=3
  wires:
  Medium/High altitude scale length/1(L_ug) -> Mux/2
  Altitude/1 -> Low altitude scale length/1(h)
  Low altitude scale length/3(L_wg) -> Mux2/1
  Low altitude scale length/2(Lvg) -> Mux1/1
  Mux1/1 -> Lvg/1
  Mux/1 -> L_ug/1
  Mux2/1 -> L_wg/1
  Medium/High altitude scale length/2(Lvg) -> Mux1/2
  Low altitude scale length/1(L_ug) -> Mux/1
  Medium/High altitude scale length/3(L_wg) -> Mux2/2

== system Quadcopter_v3_full/wind/Dryden Wind/turbulence intensities ==
  Altitude : Inport
  Windspeed at 20ft(6m) : Inport  Port=2
  High Altitude Intensity : Subsystem
  Low Altitude Intensity : Subsystem
  Mux : Mux  Inputs=2
  Mux1 : Mux  Inputs=2
  Mux2 : Mux  Inputs=2
  sigma_ug : Outport
  sigma_vg : Outport  Port=2
  sigma_wg : Outport  Port=3
  wires:
  Altitude/1 -> High Altitude Intensity/1(h), Low Altitude Intensity/1(h)
  Windspeed at 20ft(6m)/1 -> Low Altitude Intensity/2(Windspeed at 20ft(6m))
  Low Altitude Intensity/1(sigma_ug) -> Mux/1
  High Altitude Intensity/1(sigma_ug) -> Mux/2
  High Altitude Intensity/2(sigma_vg) -> Mux1/2
  Low Altitude Intensity/2(sigma_vg) -> Mux1/1
  High Altitude Intensity/3(sigma_wg) -> Mux2/2
  Low Altitude Intensity/3(sigma_wg) -> Mux2/1
  Mux1/1 -> sigma_vg/1
  Mux/1 -> sigma_ug/1
  Mux2/1 -> sigma_wg/1

== system Quadcopter_v3_full/wind/Dryden Wind/Filters on velocities2/Hu ==
  L_ug : Inport
  V : Inport  Port=2
  Noise : Inport  Port=3
  sigma_ug : Inport  Port=4
  (2/pi) : Gain  Gain=2/pi
  L_ug/V : Product  Inputs=*/
  Product : Product
  Product1 : Product
  Sqrt : Sqrt  SaturateOnIntegerOverflow=on
  Sum : Sum  Inputs=|+-
  ug_p : Integrator
  w : Product  Inputs=*/
  ugw : Outport
  wires:
  L_ug/1 -> L_ug/V/1
  V/1 -> L_ug/V/2
  L_ug/V/1 -> w/2, (2/pi)/1
  (2/pi)/1 -> Sqrt/1
  Sqrt/1 -> Product/1
  Noise/1 -> Product/2
  Product/1 -> Sum/1
  Sum/1 -> w/1
  w/1 -> ug_p/1
  ug_p/1 -> Sum/2, Product1/1
  sigma_ug/1 -> Product1/2
  Product1/1 -> ugw/1

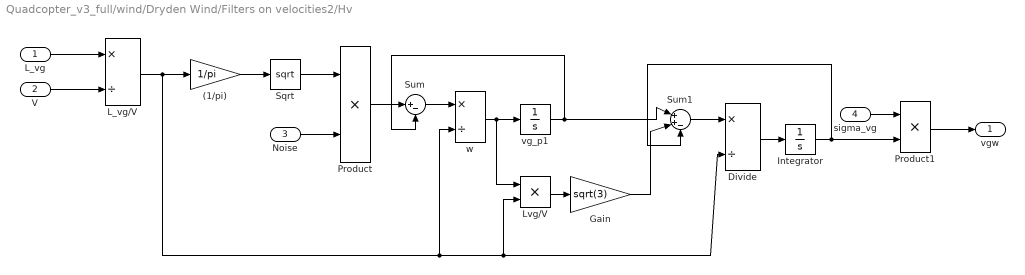
== system Quadcopter_v3_full/wind/Dryden Wind/Filters on velocities2/Hv ==
  L_vg : Inport
  V : Inport  Port=2
  Noise : Inport  Port=3
  sigma_vg : Inport  Port=4
  (1/pi) : Gain  Gain=1/pi
  Divide : Product  Inputs=*/
  Gain : Gain  Gain=sqrt(3)
  Integrator : Integrator
  L_vg/V : Product  Inputs=*/
  Lvg/V : Product
  Product : Product
  Product1 : Product
  Sqrt : Sqrt  SaturateOnIntegerOverflow=on
  Sum : Sum  Inputs=|+-
  Sum1 : Sum  Inputs=|++-
  vg_p1 : Integrator
  w : Product  Inputs=*/
  vgw : Outport
  wires:
  L_vg/1 -> L_vg/V/1
  V/1 -> L_vg/V/2
  L_vg/V/1 -> w/2, Lvg/V/2, Divide/2, (1/pi)/1
  (1/pi)/1 -> Sqrt/1
  Sqrt/1 -> Product/1
  Noise/1 -> Product/2
  Product/1 -> Sum/1
  Sum/1 -> w/1
  w/1 -> Lvg/V/1, vg_p1/1
  Lvg/V/1 -> Gain/1
  vg_p1/1 -> Sum1/1, Sum/2
  Gain/1 -> Sum1/2
  Sum1/1 -> Divide/1
  Divide/1 -> Integrator/1
  Integrator/1 -> Sum1/3, Product1/2
  Product1/1 -> vgw/1
  sigma_vg/1 -> Product1/1

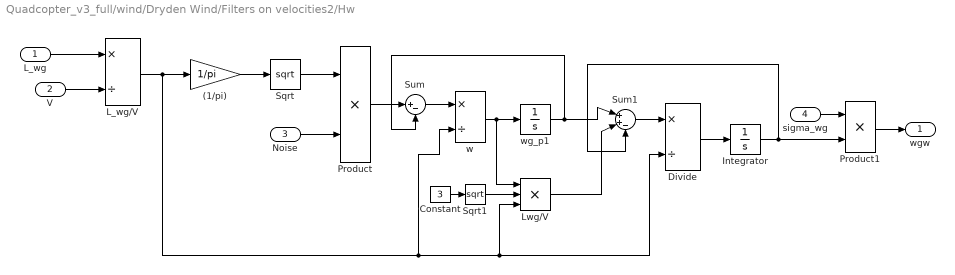
== system Quadcopter_v3_full/wind/Dryden Wind/Filters on velocities2/Hw ==
  L_wg : Inport
  V : Inport  Port=2
  Noise : Inport  Port=3
  sigma_wg : Inport  Port=4
  (1/pi) : Gain  Gain=1/pi
  Constant : Constant  Value=3
  Divide : Product  Inputs=*/
  Integrator : Integrator
  L_wg/V : Product  Inputs=*/
  Lwg/V : Product  Inputs=3
  Product : Product
  Product1 : Product
  Sqrt : Sqrt  SaturateOnIntegerOverflow=on
  Sqrt1 : Sqrt  SaturateOnIntegerOverflow=on
  Sum : Sum  Inputs=|+-
  Sum1 : Sum  Inputs=|++-
  w : Product  Inputs=*/
  wg_p1 : Integrator
  wgw : Outport
  wires:
  L_wg/1 -> L_wg/V/1
  V/1 -> L_wg/V/2
  L_wg/V/1 -> Lwg/V/3, Divide/2, w/2, (1/pi)/1
  (1/pi)/1 -> Sqrt/1
  Sqrt/1 -> Product/1
  Noise/1 -> Product/2
  Product/1 -> Sum/1
  Sum/1 -> w/1
  w/1 -> Lwg/V/1, wg_p1/1
  Lwg/V/1 -> Sum1/2
  wg_p1/1 -> Sum1/1, Sum/2
  Sum1/1 -> Divide/1
  Divide/1 -> Integrator/1
  Integrator/1 -> Product1/2, Sum1/3
  Product1/1 -> wgw/1
  sigma_wg/1 -> Product1/1
  Constant/1 -> Sqrt1/1
  Sqrt1/1 -> Lwg/V/2

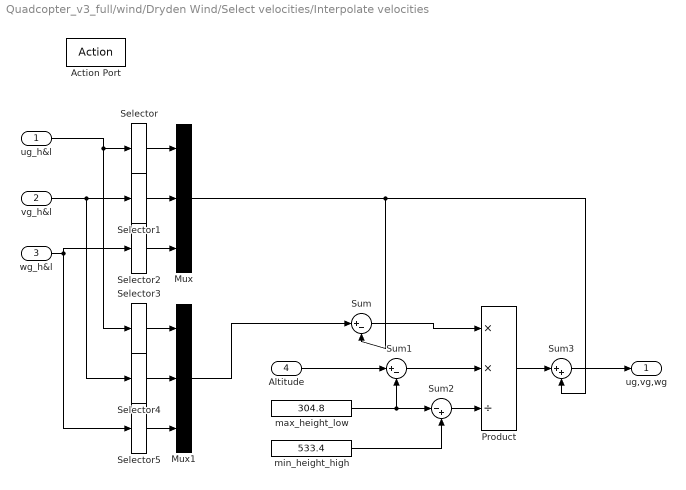
== system Quadcopter_v3_full/wind/Dryden Wind/Select velocities/Interpolate velocities ==
  ug_h&l : Inport
  vg_h&l : Inport  Port=2
  wg_h&l : Inport  Port=3
  Altitude : Inport  Port=4
  Action Port : ActionPort
  Mux : Mux  Inputs=3
  Mux1 : Mux  Inputs=3
  Product : Product  Inputs=**/
  Selector : Selector  InputPortWidth=2  IndexOptions=Index vector (dialog)  Indices=[1]  OutputSizes=1
  Selector1 : Selector  InputPortWidth=2  IndexOptions=Index vector (dialog)  Indices=[1]  OutputSizes=1
  Selector2 : Selector  InputPortWidth=2  IndexOptions=Index vector (dialog)  Indices=[1]  OutputSizes=1
  Selector3 : Selector  InputPortWidth=2  IndexOptions=Index vector (dialog)  Indices=[2]  OutputSizes=1
  Selector4 : Selector  InputPortWidth=2  IndexOptions=Index vector (dialog)  Indices=[2]  OutputSizes=1
  Selector5 : Selector  InputPortWidth=2  IndexOptions=Index vector (dialog)  Indices=[2]  OutputSizes=1
  Sum : Sum  Inputs=|+-
  Sum1 : Sum  Inputs=|+-
  Sum2 : Sum  Inputs=|-+
  Sum3 : Sum  Inputs=|++
  max_height_low : Constant  Value=304.8
  min_height_high : Constant  Value=533.4
  ug,vg,wg : Outport
  wires:
  ug_h&l/1 -> Selector3/1, Selector/1
  vg_h&l/1 -> Selector4/1, Selector1/1
  wg_h&l/1 -> Selector5/1, Selector2/1
  Selector/1 -> Mux/1
  Selector1/1 -> Mux/2
  Selector2/1 -> Mux/3
  Selector3/1 -> Mux1/1
  Selector4/1 -> Mux1/2
  Selector5/1 -> Mux1/3
  max_height_low/1 -> Sum1/2, Sum2/1
  min_height_high/1 -> Sum2/2
  Altitude/1 -> Sum1/1
  Mux1/1 -> Sum/1
  Mux/1 -> Sum3/2, Sum/2
  Sum/1 -> Product/1
  Sum1/1 -> Product/2
  Sum2/1 -> Product/3
  Product/1 -> Sum3/1
  Sum3/1 -> ug,vg,wg/1

== system Quadcopter_v3_full/wind/Dryden Wind/Select velocities/Low altitude velocities  ==
  ug_h&l : Inport
  vg_h&l : Inport  Port=2
  wg_h&l : Inport  Port=3
  Action Port : ActionPort
  Gain : Gain
  Mux : Mux  Inputs=3
  Selector : Selector  InputPortWidth=6  IndexOptions=Index vector (dialog)  Indices=[1 3 5]  OutputSizes=1
  ug,vg,wg : Outport
  wires:
  Mux/1 -> Selector/1
  ug_h&l/1 -> Mux/1
  vg_h&l/1 -> Mux/2
  wg_h&l/1 -> Mux/3
  Selector/1 -> Gain/1
  Gain/1 -> ug,vg,wg/1

== system Quadcopter_v3_full/wind/Dryden Wind/Select velocities/Medium//High altitude velocities ==
  ug_h&l : Inport
  vg_h&l : Inport  Port=2
  wg_h&l : Inport  Port=3
  Action Port : ActionPort
  Gain : Gain
  Mux : Mux  Inputs=3
  Selector : Selector  InputPortWidth=6  IndexOptions=Index vector (dialog)  Indices=[2 4 6]  OutputSizes=1
  ug,vg,wg : Outport
  wires:
  Mux/1 -> Selector/1
  ug_h&l/1 -> Mux/1
  vg_h&l/1 -> Mux/2
  wg_h&l/1 -> Mux/3
  Selector/1 -> Gain/1
  Gain/1 -> ug,vg,wg/1

== system Quadcopter_v3_full/wind/Dryden Wind/Select velocities/Merge Subsystems ==
  low : Inport
  high : Inport  Port=2
  interpolated : Inport  Port=3
  dcm : Inport  Port=4
  Demux : Demux  Outputs=3
  Merge : Merge  Inputs=3
  convert to inertial frame : MATLAB Function  TreatAsAtomicUnit=on
  ug : Outport
  vg : Outport  Port=2
  wg : Outport  Port=3
  wires:
  Merge/1 -> Demux/1
  low/1 -> Merge/1
  high/1 -> Merge/2
  interpolated/1 -> Merge/3
  Demux/1 -> convert to inertial frame/1(ug)
  Demux/2 -> convert to inertial frame/2(vg)
  Demux/3 -> convert to inertial frame/3(wg)
  convert to inertial frame/1(ugw) -> ug/1
  convert to inertial frame/2(vgw) -> vg/1
  convert to inertial frame/3(wgw) -> wg/1
  dcm/1 -> convert to inertial frame/4(dcm)

== system Quadcopter_v3_full/wind/Dryden Wind/Turbulence scale lengths/Low altitude scale length ==
  h : Inport
  Limit Function 10ft(3.048m) to 1000ft(304.8m) 1 foot = 0.3048m : Saturate  UpperLimit=304.8  LowerLimit=3.048
  Low Altitude Scale Length : Fcn  Expr=u(1)/(0.177+0.000823*u(1))^1.2
  Low Altitude Scale Length1 : Fcn  Expr=u(1)/(0.177+0.000823*u(1))^1.2
  L_ug : Outport
  Lvg : Outport  Port=2
  L_wg : Outport  Port=3
  wires:
  Low Altitude Scale Length1/1 -> Lvg/1
  Low Altitude Scale Length/1 -> L_ug/1
  h/1 -> Limit Function 10ft(3.048m) to 1000ft(304.8m) 1 foot = 0.3048m/1
  Limit Function 10ft(3.048m) to 1000ft(304.8m) 1 foot = 0.3048m/1 -> L_wg/1, Low Altitude Scale Length1/1, Low Altitude Scale Length/1

== system Quadcopter_v3_full/wind/Dryden Wind/Turbulence scale lengths/Medium//High altitude scale length ==
  Scale length at medium/high altitudes: 533.4m(1750 feet) : Constant  Value=533.4
  Scale length at medium/high altitudes: 533.4m(1750 feet)1 : Constant  Value=533.4
  Scale length at medium/high altitudes: 533.4m(1750 feet)2 : Constant  Value=533.4
  L_ug : Outport
  Lvg : Outport  Port=2
  L_wg : Outport  Port=3
  wires:
  Scale length at medium/high altitudes: 533.4m(1750 feet)/1 -> L_ug/1
  Scale length at medium/high altitudes: 533.4m(1750 feet)1/1 -> Lvg/1
  Scale length at medium/high altitudes: 533.4m(1750 feet)2/1 -> L_wg/1

== system Quadcopter_v3_full/wind/Dryden Wind/turbulence intensities/High Altitude Intensity ==
  note: (feet)----(m)
      | 500---154.2
      | 1750--- 539.7
      | 3750--- 1156.5
      | 7500--- 2313
      | 15000--- 4626
      | 25000--- 7710
      | 35000--- 10794
      | 45000--- 13878
      | 55000--- 16962
      | 65000--- 20046
      | 75000--- 23130
      | 80000--- 24672
  h : Inport
  Interpolation Using Prelookup : Interpolation_n-D  Table=[3.2,4.2,6.6,8.6,11.8,15.6,18.7;2.2,3.6,6.9,9.6,13,17.6,21.5;1.5,3.3,7.4,10.6,16,23,28.4;0,1.6,6.7,10.1,15.1,23.6,30.2;0,0,4.6,8,11.6,22.1,30.7;0,0,2.7,6.6,9.7,20,31;0,0,0.4,5,8.1,16,25.2;0,0,0,4.2,8.2,15.1,23.1;0,0,0,2.7,7.9,12.1,17.5;0,0,0,0,4.9,7.9,10.7;0,0,0,0,3.2,6.2,8.4;0,0,0,0,2.1,5.1,7.2]  InternalRulePriority=Speed
  Prelookup Index Search (altitude) : PreLookup  BreakpointsData=[154.2;539.7;1156.5;2313;4626;7710;10794;13878;16962;20046;23130;24672]  BeginIndexSearchUsingPreviousIndexResult=on  UseLastBreakpoint=on
  Prelookup Index Search (prob of exceed) : PreLookup  BreakpointsData=[1:7]  BeginIndexSearchUsingPreviousIndexResult=on  UseLastBreakpoint=on
  Probability of Exceedance : Constant  Value=4
  Scope{,1..4} (5 alike) : Scope
  sigma_ug : Outport
  sigma_vg : Outport  Port=2
  sigma_wg : Outport  Port=3
  wires:
  Probability of Exceedance/1 -> Prelookup Index Search (prob of exceed)/1
  Prelookup Index Search (prob of exceed)/1 -> Scope/1, Interpolation Using Prelookup/3
  Prelookup Index Search (prob of exceed)/2 -> Scope1/1, Interpolation Using Prelookup/4
  Prelookup Index Search (altitude)/2 -> Scope3/1, Interpolation Using Prelookup/2
  h/1 -> Prelookup Index Search (altitude)/1
  Prelookup Index Search (altitude)/1 -> Interpolation Using Prelookup/1, Scope2/1
  Interpolation Using Prelookup/1 -> sigma_wg/1, sigma_vg/1, Scope4/1, sigma_ug/1

== system Quadcopter_v3_full/wind/Dryden Wind/turbulence intensities/Low Altitude Intensity ==
  h : Inport
  Windspeed at 20ft(6m) : Inport  Port=2
  Gain : Gain  Gain=0.1
  Limit Height h<304.8m(1000ft) : Saturate  UpperLimit=304.8  LowerLimit=0
  Low Altitude Intensity : Fcn  Expr=1/(0.177+0.000823*u(1))^0.4
  Product : Product
  Product1 : Product
  sigma_ug : Outport
  sigma_vg : Outport  Port=2
  sigma_wg : Outport  Port=3
  wires:
  Gain/1 -> sigma_wg/1, Product1/2, Product/2
  Low Altitude Intensity/1 -> Product1/1, Product/1
  Limit Height h<304.8m(1000ft)/1 -> Low Altitude Intensity/1
  Product1/1 -> sigma_vg/1
  Product/1 -> sigma_ug/1
  Windspeed at 20ft(6m)/1 -> Gain/1
  h/1 -> Limit Height h<304.8m(1000ft)/1

== matlab function Quadcopter_v3_full/wind/LES_wind/MATLAB Function ==
  data: x input; wind_vel output; t input; u_wind input; v_wind input; w_wind input; P parameter
function wind_vel = spa_temp(x,t,u_wind,v_wind,w_wind,P)
%% extract wind from the wind grid given current simulation time and states


wind_vel=zeros(1,3);
coder.extrinsic("griddedInterpolant")
res = P.res;

%sometimes z goes positive down so making it positive
if x(3)>0
    x(3)=0;
    elseif x(3)<0 %z is positive down but wind_z positive up so taking the abs
        x(3)=abs(x(3));
end

idx_num = [x(3)/res(3) x(2)/res(2) x(1)/res(1)]+ ones(1,3); %because wind data doesnot start at 0,so shifting to start after 1m
% idx_num = [x(3) x(2) x(1)];
%  idx=round(idx_num)+1;
% t=round(t);

if t <1
    t=1+t;
end



point_q=[t,idx_num];
% disp(point_q)
F_u = griddedInterpolant(u_wind);
F_v = griddedInterpolant(v_wind);
F_w = griddedInterpolant(w_wind);

wind_vel=double([F_u(point_q) F_v(point_q) F_w(point_q)]);%w is positive in LES wind
end

== matlab function Quadcopter_v3_full/Estimator/sensors/gps ==
  settings: updateMethod=DISCRETE
  data: x input; GPS output; P parameter
function GPS  = fcn(x,P)
%#codegen
Pn = x(1);
Pe = x(2);
Pd = x(3);

%% model1 
bias_gps_x=P.bias_gps_x;
bias_gps_y=P.bias_gps_y;
bias_gps_z=P.bias_gps_z;
sigma_gps=P.sigma_gps;
Pn = Pn + bias_gps_x + sigma_gps*randn;
Pe = Pe + bias_gps_y + sigma_gps*randn;
Pd = Pd + bias_gps_z + sigma_gps*randn;
GPS=[Pn;Pe;Pd];
%% model2
%     % GPS parameters
%     Ts_gps = 1; % sample rate of GPS in s
%     beta_gps = 1/1100; % 1/s
%     sigma_n_gps = 0.21;
%     sigma_e_gps = 0.21; 
%     sigma_h_gps = 0.40;
%     % persistent variables that define random walk of GPS sensors
%     persistent eta_n;
%     persistent eta_e;
%     persistent eta_h;
%     
%     
%     if t==0  % initialize persistent variables
%         eta_n = 0;
%         eta_e = 0;
%         eta_h = 0;
%     else      % propagate persistent variables
%         eta_n = exp(beta_gps*Ts_gps)*eta_n + sigma_n_gps*randn;
%         eta_e = exp(beta_gps*Ts_gps)*eta_e + sigma_e_gps*randn;
%         eta_h = exp(beta_gps*Ts_gps)*eta_h + sigma_h_gps*randn;
%     end
%     
%     % construct North, East, and altitude GPS measurements
%     y_gps_n = Pn + eta_n;
%     y_gps_e = Pe + eta_e; 
%     y_gps_h = Pd + eta_h; 
%     
%     GPS=[y_gps_n;y_gps_e;y_gps_h];

end

== matlab function Quadcopter_v3_full/Control Gate ==
  data: t input; u input; U_final output; u_adjusted input
function U_final = gate(t,u,u_adjusted)


if t<0   %for spatial temporal wind BMET may not work during initial take off, so change time to t=4 sec
    U_final=u;
else
    flag = isnan(u_adjusted);

    if any(flag==1) ||u_adjusted(1) < 0
        U_final = u;
    else

          U_final = u_adjusted;
    end


end
end

== matlab function Quadcopter_v3_full/Controller /High Level Controller/RS Controller ==
  data: x input; r input; y output; P parameter; t input
function y  = MCV(x, r, P,t)
%Risk Sensitive Control 

  %inputs
  %x---states; this will give all states, f_c and omega
  %prev_state---states from last time step
  %sumError-- not need
  %ref--- reference


xref= r(1:10);
x_c=x(1:10);

sol = P.Soln;
time=[sol(1,:).t];
  
idxA=find(time>=t);
idx=idxA(1);
K0=sol(idx).K;
y=(K0*(x_c-xref));  %desired omegas and fc

%10/20/2021 added by hao
if abs(y(1))>pi/2
    y(1) = (pi/2)*sign(y(1));
end 
if abs(y(2))>pi/2
    y(2) = (pi/2)*sign(y(2));
end 
if abs(y(3))>pi/2
    y(3) = (pi/2)*sign(y(3));
end 
end

== matlab function Quadcopter_v3_full/Controller /High Level Controller/trajectory/circle_traj ==
  settings: updateMethod=DISCRETE
  data: X input; y output
function y = fcn(X)
%states
Pn=X(1);
Pe=X(2);
Pd=X(3);
P=[Pn;Pe;Pd];

theta = 1:30:360;
x0 = 100;
y0 = 100;
r = 100;
Pn = x0 + r*cosd(theta);
Pe = y0 + r*sind(theta);
Pd = -100;

persistent k;
if isempty(k)
    k = 1;
end
P_d=[Pn(k);Pe(k);Pd];
if norm(P_d-P) < 10
   k=k+1;
end

y = [P_d(1);P_d(2);P_d(3);0;0;0;0;0;0;0;0;0];
end

== matlab function Quadcopter_v3_full/Controller /High Level Controller/trajectory/squre_traj ==
  settings: updateMethod=DISCRETE
  data: X input; y output
function y = fcn(X)
%states
Pn=X(1);
Pe=X(2);
Pd=X(3);
P=[Pn;Pe;Pd];

% Pn_d = [50;100;100;50;50];
% Pe_d = [50;50;100;100;50];
% Pd_d = [-50;-50;-50;-50;-50];
% yaw_d = [0.7854;1.5708;0;-1.5708;-3.14];

Pn_d = [100;200;200;100;100];
Pe_d = [100;100;200;200;100];
Pd_d = [-8;-8;-8;-8;-8];
% Pd_d = [-50;-50;-50;-50;-50];
% yaw_d = [-0.7854;-1.5708;0;1.5708;3.14];
yaw_d = [0;0;0;0;0];
persistent k;
if isempty(k)
    k = 1;
end
P_d=[Pn_d(k);Pe_d(k);Pd_d(k)];
psi_d= yaw_d(k);
if norm(P_d-P) < 10 && k<5
   k=k+1;
end

y = [P_d(1);P_d(2);P_d(3);0;0;0;0;0;psi_d;0;0;0;0;0];%increase it to match
end

== matlab function Quadcopter_v3_full/Controller /Low-Level Controller/Low level controller ==
  data: true_u input; u output; desired input; P parameter
function u = fd(true_u, desired,P)
%References: Dynamics using Quaternion for full-state feedback control
%adapted from "Onboard State Dependent LQR for Agile Quadrotors"
%see "AIAA paper draft for full model"

  %inputs
  %prevwb--- current omega
  %desired-desired(1)-desired wx
         %-desired(2)-desired wy
         %-desired(3)-desired wz
         %-desired(4)-desired fc
Ix = P.Ix;
Iy = P.Iy;
Iz = P.Iz;
J=[Ix , 0 , 0;
    0 , Iy , 0;
    0 , 0  , Iz];

P_g=diag([70,70,.001]);
des_wb=desired(1:3);
prev_wb=true_u(1:3);

tau= J*P_g*(des_wb-prev_wb)+ cross(prev_wb,J*prev_wb);

u=[ desired(4),tau'];


end
